simulink model "PID"  (R2018b)
settings: Solver=VariableStepAuto  StartTime=0.0  StopTime=7  RelTol=1e-3
values from neighbouring files (symbols this model uses):
  Law = [kp, kd]    [Init.m]    (also in LAUNCH_Backstepping.m = [lambda, kd]; LAUNCH_Backstepping_adapt.m; LAUNCH_CToque.m; WS_regressor.mat = [500 50])
  param = param'    [Init.m]    (also in WS_regressor.mat = [1 1 1 1 1 1 0 1 1 1 3 3 ... (14 elements, 7x2)])
  pulsazione_circolare = 1    [Init.m]    (also in WS_regressor.mat)
  x0 = -1.5    [Init.m]    (also in WS_regressor.mat)
  y0 = 2    [Init.m]    (also in WS_regressor.mat)
undefined symbols (not defined in the file or in its folder): A_circolare, cond_iniziali
libraries: simulink x1
settings Model: Creator=AmatoPi  LastModifiedBy=AmatoPi

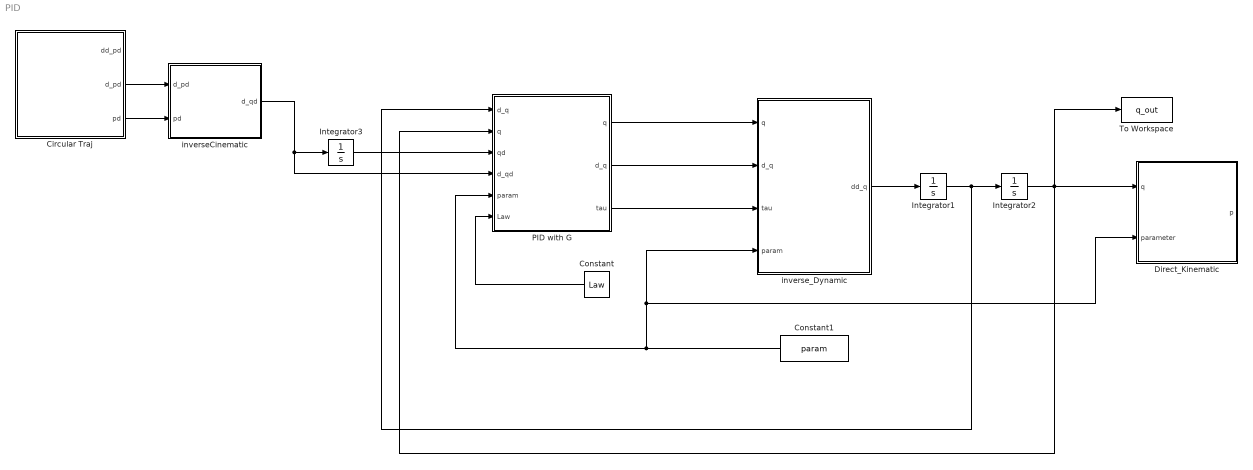
== system PID ==
  Circular Traj : Subsystem
  Constant : Constant  Value=Law
  Constant1 : Constant  Value=param
  Direct_Kinematic : MATLAB Function  TreatAsAtomicUnit=on
  Integrator1 : Integrator  InitialCondition=[0;0;0;0;0;0]
  Integrator2 : Integrator  InitialCondition=cond_iniziali
  Integrator3 : Integrator  InitialCondition=[0;0;0;0;0;0]
  PID with G : MATLAB Function  TreatAsAtomicUnit=on
  To Workspace : ToWorkspace  VariableName=q_out  SaveFormat=Timeseries  SampleTime=-1
  inverseCinematic : MATLAB Function  TreatAsAtomicUnit=on
  inverse_Dynamic : MATLAB Function  TreatAsAtomicUnit=on
  wires:
  Circular Traj/3(pd) -> inverseCinematic/2(pd)
  Circular Traj/2(d_pd) -> inverseCinematic/1(d_pd)
  PID with G/3(tau) -> inverse_Dynamic/3(tau)
  PID with G/2(d_q) -> inverse_Dynamic/2(d_q)
  PID with G/1(q) -> inverse_Dynamic/1(q)
  inverse_Dynamic/1(dd_q) -> Integrator1/1
  Integrator1/1 -> PID with G/1("d_q "), Integrator2/1
  Integrator2/1 -> Direct_Kinematic/1(q), To Workspace/1, PID with G/2("q ")
  Constant/1 -> PID with G/6(Law)
  Constant1/1 -> PID with G/5(param), Direct_Kinematic/2(parameter), inverse_Dynamic/4(param)
  inverseCinematic/1(d_qd) -> PID with G/4(d_qd), Integrator3/1
  Integrator3/1 -> PID with G/3(qd)

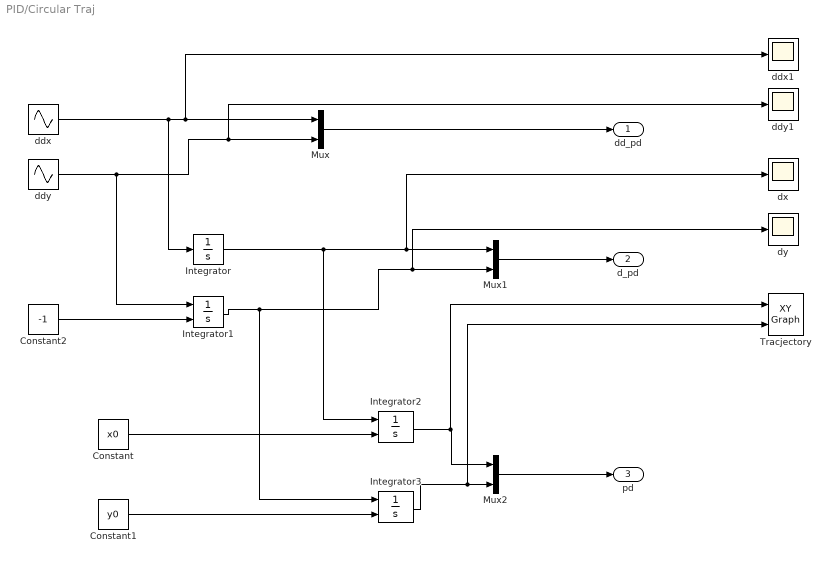
== system PID/Circular Traj ==
  Constant : Constant  Value=x0
  Constant1 : Constant  Value=y0
  Constant2 : Constant  Value=-1
  Integrator : Integrator
  Integrator1 : Integrator  InitialConditionSource=external
  Integrator2 : Integrator  InitialConditionSource=external
  Integrator3 : Integrator  InitialConditionSource=external
  Mux : Mux  Inputs=2
  Mux1 : Mux  Inputs=2
  Mux2 : Mux  Inputs=2
  Tracjectory : simulink/Sinks/XY Graph  xmin=xL  xmax=xR  ymin=yD  ymax=yU  st=-1
  ddx : Sin  Amplitude=A_circolare  Frequency=pulsazione_circolare  Phase=pi/2  SampleTime=0
  ddx1 : Scope
  ddy : Sin  Amplitude=A_circolare  Frequency=pulsazione_circolare  SampleTime=0
  ddy1 : Scope
  dx : Scope
  dy : Scope
  dd_pd : Outport
  d_pd : Outport  Port=2
  pd : Outport  Port=3
  wires:
  Mux/1 -> dd_pd/1
  ddx/1 -> Integrator/1, ddx1/1, Mux/1
  ddy/1 -> ddy1/1, Mux/2, Integrator1/1
  Mux1/1 -> d_pd/1
  Integrator2/1 -> Tracjectory/1, Mux2/1
  Mux2/1 -> pd/1
  Integrator/1 -> Integrator2/1, dx/1, Mux1/1
  Integrator3/1 -> Tracjectory/2, Mux2/2
  Integrator1/1 -> Integrator3/1, dy/1, Mux1/2
  Constant/1 -> Integrator2/2
  Constant1/1 -> Integrator3/2
  Constant2/1 -> Integrator1/2

== matlab function PID/PID with G ==
  data: q output; d_q output; d_q input; tau output; q input; qd input; d_qd input; param input; Law input
function [q,d_q,tau]  = PID_Contro(d_q, q, qd, d_qd, param, Law)

    kp = Law(1).*eye(6);
    kd = Law(2).*eye(6);
    [~,~,G] = Dinamica(param,q,dq);
    
    error = qd - q;
    d_error = d_qd - d_q;
    
    tau = kp*error + kd*d_error + G;
    
end

== matlab function PID/inverseCinematic ==
  data: d_pd input; pd input; d_qd output
function d_qd = inverseCin(d_pd,pd)

    d_qd = zeros(3,1);

end

== matlab function PID/inverse_Dynamic ==
  data: q input; dd_q output; d_q input; tau input; param input
function dd_q = inverseDynamic(q,d_q,tau,param)
    
    [B,C,G] = Dinamica(param,q,dq);

    tot = Tau - C*dq - G;    
    ddq = B\(tot);

end

== matlab function PID/Direct_Kinematic ==
  data: q input; p output; parameter input
function p = DirectK(q,parameter)

	[p,com,head] = Direct_Kinematics(parameter,q);
    
    

end
